simulink library "PowerFlowLib2013amdl"  (Simulink 8.1)
settings: Solver=ode45  StartTime=0.0  StopTime=10.0  RelTol=1e-3
undefined symbols (not defined in the file or in its folder): AirProp, C, F1, Fanmap, Fld1, Fld2, fueltankdata, HydProp, HydraulicLoad, IBFD_exc, L, LoadFluidProps, magnitude, MSSN, n_alghts, PumpProp, pwr_alghts, R_fd_exc, Rcore, Ts, VBFD_exc
libraries: PowerFlowLib x32, simulink x14, powerlib_extras x2, dspstat3 x2
(part 4 of 11)

== system PowerFlowLib2013amdl/Energy & Power Systems/Additional Systems ==
  Commercial Cabin Systems : Subsystem  mask(Commercial Cabin Systems){n_pax=150, n_sockets=3, n_oven=4, pwr_oven=3800, pf_oven=.707, q_oven=95, n_bev=3, pwr_bev=3800, pf_bev=.707, q_bev=95, n_rlghts=150, pwr_rlghts=5, q_rlghts=95, n_clghts=20, pwr_clghts=15, q_clghts=95, n_IFE=150, pwr_IFE=25}
      mask prompts: n_pax "Seating Capacity"; n_sockets "Number of Electrical Sockets in Cabin"; n_oven "Number of Ovens"; pwr_oven "Nominal Power [W]"; pf_oven "Power Factor"; q_oven "Heat Loss Output [W]"; n_bev "Number of Beverage Makers"; pwr_bev "Nominal Power [W]"; pf_bev "Power Factor"; q_bev "Heat Loss Output [W]"; n_rlghts "Number of Reading Lights"; pwr_rlghts "Power Consumption per Lamp [W]"; q_rlghts "Heat Loss Output [W]"; n_clghts "Number of Cabin Lights"; pwr_clghts "Power Consumption per Light [W]"; q_clghts "Heat Loss Output [W]"; n_IFE "Individual Seat Models"; pwr_IFE "Power Consumption per Seat Model [W]"
      mask help:
      | Calculation of galley electrical loads, cabin lighting loads, and in-flight entertainment (IFE) electrical loads.
      |
      | Input to the block requires the mission profile for determination of usage and cyclical loading.
  External Lights : Subsystem  mask(Commercial Cabin Systems){n_pax=150, n_sockets=3, n_oven=4, pwr_oven=3800, pf_oven=.707, q_oven=95, n_bev=3, pwr_bev=3800, pf_bev=.707, q_bev=95, n_rlghts=150, pwr_rlghts=5, q_rlghts=95, n_clghts=20, pwr_clghts=15, q_clghts=95, n_IFE=150, pwr_IFE=25}
      mask prompts: n_pax "Seating Capacity"; n_sockets "Number of Electrical Sockets in Cabin"; n_oven "Number of Ovens"; pwr_oven "Nominal Power [W]"; pf_oven "Power Factor"; q_oven "Heat Loss Output [W]"; n_bev "Number of Beverage Makers"; pwr_bev "Nominal Power [W]"; pf_bev "Power Factor"; q_bev "Heat Loss Output [W]"; n_rlghts "Number of Reading Lights"; pwr_rlghts "Power Consumption per Lamp [W]"; q_rlghts "Heat Loss Output [W]"; n_clghts "Number of Cabin Lights"; pwr_clghts "Power Consumption per Light [W]"; q_clghts "Heat Loss Output [W]"; n_IFE "Individual Seat Models"; pwr_IFE "Power Consumption per Seat Model [W]"
      mask help:
      | Calculation of galley electrical loads, cabin lighting loads, and in-flight entertainment (IFE) electrical loads.
      |
      | Input to the block requires the mission profile for determination of usage and cyclical loading.

== system PowerFlowLib2013amdl/Energy & Power Systems/Electrical ==
  Battery : Subsystem
  Converters : Subsystem
  Coordinate Transformation : Subsystem
  Inverters : Subsystem
  Loads : Subsystem
  Loss Estimation : Subsystem
  Machines : Subsystem
  Rectifiers : Subsystem
  Systems : Subsystem

== system PowerFlowLib2013amdl/Energy & Power Systems/Hydraulic ==
  Bypass Valve : Subsystem  mask(Bypass Valve){}
      mask help:
      | Calculates hydraulic fluid bypass.
      |
      | Flow Out - hydraulic fluid flow to the actuators.
      | Bypass - hydraulic fluid flow back to the reservoir.
      mask Display:
      | port_label('input',1,'{\bf Flow In}','TexMode','on')
      | port_label('input',2,'{\bf Req Flow}','TexMode','on')
      | 
      | port_label('output',1,'{\bf Flow Out}','TexMode','on')
      | port_label('output',2,'{\bf Bypass}','TexMode','on')
  Engine Driven Pump : Subsystem  mask(Engine Driven Hydraulic Pump){RPM=3750, disp=39, eta_mech=95, eta_v=85, nom_T=40, nom_w=393, nom_delP=20684}
      mask prompts: RPM "Fixed RPM"; disp "Fixed Displacement [cm³/rev]"; eta_mech "Mechanical Efficiency [%]"; eta_v "Volumetric Efficiency [%]"; nom_T "Nominal Fluid Temperature [°C]"; nom_w "Nominal Angular Velocity [rad/s]"; nom_delP "Nominal Pressure Differential [kPa]"
      mask help:
      | This is a fixed displacement, uni-directional hydraulic pump.  Flow rate is calculated by this block.  Pressure up-stream and down-stream are required inputs.
      |
      | Block Inputs
      | #1: Hydraulic fluid properties from reservoir
      | #2: Shaft RPM from aux. gear box
      | #3: Upstream system hydraulic pressure [kPa]
      |
      | Block Outputs
      | #1: Fluid properties
      | #2: Shaft torque applied to aux. gear box [Nm]
      mask Callback eta_mech:
      | h      = get_param(gcb,'handle');   % Get block handle
      | hblock = get(h);                    % Parse out handles structure
      | 
      | if str2num(hblock.eta_mech) == 0
      |     set_param(gcb,'eta_mech','100')
      | elseif str2num(hblock.eta_mech) < 1
      |     set_param(gcb,'eta_mech',num2str(str2num(hblock.eta_mech)*100))
      | elseif str2num(hblock.eta_mech) > 100
      |     set_param(gcb,'eta_mech',num2str(100))
      | end
      | 
      | clear h hblock
      mask Callback eta_v:
      | h      = get_param(gcb,'handle');   % Get block handle
      | hblock = get(h);                    % Parse out handles structure
      | 
      | if str2num(hblock.eta_v) == 0
      |     set_param(gcb,'eta_v','100')
      | elseif str2num(hblock.eta_v) < 1
      |     set_param(gcb,'eta_v',num2str(str2num(hblock.eta_v)*100))
      | elseif str2num(hblock.eta_v) > 100
      |     set_param(gcb,'eta_v',num2str(100))
      | end
      | 
      | clear h hblock
      mask Display:
      | image(imread('hyd_edp_fixed.png'))
      | 
      | port_label('input',1,'{\bf Flow In}','TexMode','on')
      | port_label('input',2,'{\bf Shaft RPM}','TexMode','on')
      | port_label('input',3,'{\bf System Pressure (kPa)}','TexMode','on')
      | 
      | port_label('output',1,'{\bf Flow Out}','TexMode','on')
      | port_label('output',2,'{\bf Shaft Torque (Nm)}','TexMode','on')
  Fluid Reservoir : Subsystem  mask(Fluid Reservoir){res_vol=.25, bleed_flowrate=.05, pres_loss=1, T_init=300, P_init=1500, mass_init=30}
      mask prompts: res_vol "Resevoir Volume [m³]"; bleed_flowrate "Max Bleed Air Supply Rate [kg/s]"; pres_loss "Air Pressure Losses [%]"; T_init "Initial Fluid Temp [K]"; P_init "Initial Air Pressure [kPa]"; mass_init "Initial Fluid Mass [kg]"
      mask help:
      | Block Inputs
      | #1: Bleed air properties (Bus signal)
      | #2: Bypass return from bypass valve
      | #3: Mass flow rate pumped out by hydraulic pump
      | #4: Mass flow rate returned from actuators
      |
      | Block Outputs
      | #1: Bleed air demanded to maintain pressurization
      | #2: Hydraulic fluid properties in the reservoir
      mask Display:
      | image(imread('hyd_res.png'))
      | 
      | port_label('input',1,'{\bf Bleed In}','TexMode','on')
      | port_label('input',2,'{\bf Bypass Return}','TexMode','on')
      | port_label('input',3,'{\bf m_d_o_t Out}','TexMode','on')
      | port_label('input',4,'{\bf m_d_o_t Return}','TexMode','on')
      | 
      | port_label('output',1,'{\bf Bleed Demand}','TexMode','on')
      | port_label('output',2,'{\bf Fluid Out}','TexMode','on')
  Hydraulic Load : Subsystem  mask(Hydraulic Loading){fileslct=off, filename=HydraulicLoad.mat, filedir=C:\Users\mwillms4\Dropbox\School\Graduate\Research\PowerFlow Development\PowerFlow Summer 2013\PropertyTables\HydraulicLoad.mat, var_struct=HydraulicLoad, h_load=B_737 - rudder}
      mask prompts: fileslct "Select Hydraulic Load File?"; filename "Hydraulic Load File"; filedir "Hydraulic Load File Location"; var_struct "Structure Name (in workspace)"; h_load "Hydraulic Load"
      mask init:
      | h      = get_param(gcb,'handle');   % Get block handle
      | blk    = gcb; 
      | hblock = get(h);
      | 
      | set_param(blk,'fileslct','off');     % turn off manual switch
      | 
      | [platform,load] = strtok(hblock.h_load,' - ');
      | set_param([blk,'/m_dot'],'Table',[hblock.var_struct,'.',platform,'.',load(4:size(load,2))]);
      | 
      | [a,b] = size(evalin('base',[hblock.var_struct,'.',platform,'.',load(4:size(load,2))]));
      | 
      | set_param([blk,'/m_dot'],'BreakpointsForDimension1',['[1:',num2str(a),']']);
      | set_param([blk,'/m_dot'],'BreakpointsForDimension2',['[0:',num2str(b-1),']']);
      | 
      | clear h blk hblock a b platform load
      mask Callback fileslct:
      | h      = get_param(gcb,'handle');   % Get block handle
      | blk    = gcb;
      | hblock = get(h);     % Parse out handles structure
      | 
      | 
      | if strcmp(hblock.fileslct,'on') == 1;
      |     RR_SetPerfSlct(2,0);                    % call uiopen script
      |     set_param(blk,'fileslct','off');     % turn off manual switch
      | 
      |     hblock = get(h);
      | 
      |     s = whos('-FILE',hblock.filedir);
      |     if exist(s.name) == 1
      |         error(['Variable ',s.name,' already exists in the Workspace. Unable to load ',hblock.filename])
      |     end
      | end
      | 
      | clear h blk hblock s
      mask TypeOptions h_load: B_737 - rudder | B_737 - ailerons | B_737 - landing_gear | B_737 - elevator | B_737 - thrust_rev | Emb_145 - rudder | Emb_145 - ailerons | Emb_145 - landing_gear | Emb_145 - elevator | Emb_145 - thrust_rev
      mask Callback h_load:
      | h      = get_param(gcb,'handle');   % Get block handle
      | blk    = gcb;
      | hblock = get(h);     % Parse out handles structure
      | 
      | if strcmp('0',hblock.filename) ~= 1
      |     s = whos('-FILE',hblock.filename);
      | 
      |     while strcmp('<no load>',hblock.h_load) == 1
      | 
      |         hydr = fieldnames(eval(s.name));
      |         for i = 1:size(hydr,1)
      |             hydr_load = fieldnames(getfield(HydraulicLoad,hydr{i}));
      |             for j = 1:size(hydr_load,1);
      |                if ((j==1) && (i==1))
      |                     hydstr_ld = [hydr{i},' - ',hydr_load{j}];
      |                else
      |                     hydstr_ld = strcat(hydstr_ld,char(124),[hydr{i},' - ',hydr_load{j}]);
      |                end
      |             end
      |         end
      | 
      |         % Get the mask parameter values. This is a cell array of strings.
      |         styl = get_param(blk,'MaskStyles');
      |         vis = get_param(blk,'MaskVisibilities');
      |         str = get_param(blk,'MaskPromptString');
      | 
      |         % fill the mask with the parameters
      |         set_param(blk,'MaskVisibilities',vis,'MaskPromptString',str,'MaskStyles',[styl(1:3);strcat('popup(',hydstr_ld,')');styl(5)]);
      | 
      |         hblock = get(h);     % Parse out handles structure
      |     end
      | 
      | 
      | end
      | clear s h blk hblock styl vals vis str pmpstr i indx pumps hydstr hydr j
      mask Display:
      | port_label('input',1,'{\bf Flow In}','TexMode','on')
      | port_label('input',2,'{\bf Flight Phase}','TexMode','on')
      | 
      | port_label('output',1,'{\bf Return}','TexMode','on')
      | port_label('output',2,'{\bf Power}','TexMode','on')
      | 
      | text(0.5,0.9,get_param(gcb,'h_load'),'horizontalAlignment','center')

== system PowerFlowLib2013amdl/Energy & Power Systems/Thermal ==
  Anti-Ice : Subsystem  mask(Anti-Ice System){ice_sys=Wing, E_src=Electrical, dfine=off, pwr=0, m_dot=0}
      mask prompts: ice_sys "Anti-Ice System"; E_src "Energy Source"; dfine "Define Energy Consumption Externally?"; pwr "Power Consumption [kW]"; m_dot "Bleed Air Flow Rate [kg/s]"
      mask help:
      | Simulates power lost due to anti-ice systems.
      |
      | Block Inputs:
      | 1. On/Off Control Input (1/0 for On/Off)
      | 2. Power/Flow Rate Consumption (optional)
      | Note: Keep units as kg/s or kW
      |
      | Block Outputs:
      | 1. Demanded Electrical Power or Mass Flow Rate
      mask init:
      | h      = get_param(gcb,'handle');   % Get block handle
      | blk    = gcb; 
      | hblock = get(h);     % Parse out handles structure 
      | 
      | if strcmp('on',hblock.dfine) == 1;
      |     
      | else
      |     
      |     if strcmp('Engine Bleed Air',hblock.E_src) == 1;
      |         set_param([gcb,'/Load'],'Value',hblock.m_dot)
      |     elseif strcmp('APU Bleed Air',hblock.E_src) == 1;
      |         set_param([gcb,'/Load'],'Value',hblock.m_dot)
      |     elseif strcmp('Pneumatic Manifold',hblock.E_src) == 1;
      |         set_param([gcb,'/Load'],'Value',hblock.m_dot)
      |     elseif strcmp('Electrical',hblock.E_src) == 1;
      |         set_param([gcb,'/Load'],'Value',hblock.pwr)
      |     else
      |         msgbox(['Incorrect setting for Energy Source in ',hblock.Name]);
      |     end
      |         
      | end
      | 
      | 
      | try
      |     delete_line(blk,'LoadSwitch/1','LoadBus/1');
      | end
      | 
      | linehandle = add_line(blk,'LoadSwitch/1','LoadBus/1');
      | 
      | if strcmp('Engine Bleed Air',hblock.E_src) == 1;
      |     set(linehandle,'name','mdot_kgps');
      | elseif strcmp('APU Bleed Air',hblock.E_src) == 1;
      |     set(linehandle,'name','mdot_kgps');
      | elseif strcmp('Pneumatic Manifold',hblock.E_src) == 1;
      |     set(linehandle,'name','mdot_kgps');
      | elseif strcmp('Electrical',hblock.E_src) == 1;
      |     set(linehandle,'name','pwr_kW');
      | else
      |     msgbox(['Incorrect setting for Energy Source in ',hblock.Name]);
      | end
      | 
      | 
      | 
      | 
      | clear h blk hblock
      mask TypeOptions ice_sys: Engine Cowl | Wing
      mask TypeOptions E_src: Engine Bleed Air | APU Bleed Air | Pneumatic Manifold | Electrical
      mask Callback E_src:
      | h      = get_param(gcb,'handle');   % Get block handle
      | blk    = gcb;
      | hblock = get(h);     % Parse out handles structure
      | 
      | vis = get_param(blk,'MaskVisibilities');
      | if strcmp('on',hblock.dfine) == 0;
      |     if strcmp('Engine Bleed Air',hblock.E_src) == 1;
      |         set_param(blk,'MaskVisibilities',{vis{1};vis{2};vis{3};'off';'on'}) % set visibility
      |     elseif strcmp('APU Bleed Air',hblock.E_src) == 1;
      |         set_param(blk,'MaskVisibilities',{vis{1};vis{2};vis{3};'off';'on'}) % set visibility
      |     elseif strcmp('Pneumatic Manifold',hblock.E_src) == 1;
      |         set_param(blk,'MaskVisibilities',{vis{1};vis{2};vis{3};'off';'on'}) % set visibility
      |     elseif strcmp('Electrical',hblock.E_src) == 1;
      |         set_param(blk,'MaskVisibilities',{vis{1};vis{2};vis{3};'on';'off'}) % set visibility
      |     else
      |         msgbox(['Incorrect setting for Energy Source in ',hblock.Name]);
      |     end
      | end
      | 
      | clear h blk hblock vis
      mask Callback dfine:
      | h      = get_param(gcb,'handle');   % Get block handle
      | blk    = gcb;
      | hblock = get(h);     % Parse out handles structure
      | 
      | vis = get_param(blk,'MaskVisibilities');
      | 
      | if strcmp('on',hblock.dfine) == 1;
      |     try
      |         add_block('simulink/Sources/In1',[blk,'/Value'],'Position',[30,30,60,43]);
      |         delete_unconnected_lines();
      |         add_line(blk,'Value/1','Switch1/1');
      |     end
      |     set_param([blk,'/External Define'],'Value','1');
      |     set_param(blk,'MaskVisibilities',{vis{1};vis{2};vis{3};'off';'off'})
      | else
      |     set_param([blk,'/External Define'],'Value','0');
      |     try
      |         delete_block([blk,'/Value']);
      |     end
      |     if strcmp('Engine Bleed Air',hblock.E_src) == 1;
      |         set_param(blk,'MaskVisibilities',{vis{1};vis{2};vis{3};'off';'on'}) % set visibility
      |     elseif strcmp('APU Bleed Air',hblock.E_src) == 1;
      |         set_param(blk,'MaskVisibilities',{vis{1};vis{2};vis{3};'off';'on'}) % set visibility
      |     elseif strcmp('Pneumatic Manifold',hblock.E_src) == 1;
      |         set_param(blk,'MaskVisibilities',{vis{1};vis{2};vis{3};'off';'on'}) % set visibility
      |     elseif strcmp('Electrical',hblock.E_src) == 1;
      |         set_param(blk,'MaskVisibilities',{vis{1};vis{2};vis{3};'on';'off'}) % set visibility
      |     else
      |         msgbox(['Incorrect setting for Energy Source in ',hblock.Name]);
      |     end
      | end
      | 
      | clear h blk hblock vis
      mask Display:
      | h      = get_param(gcb,'handle');   % Get block handle
      | blk    = gcb;
      | hblock = get(h);     % Parse out handles structure
      | 
      | text(0.5,0.9,['Source: ',hblock.E_src],'HorizontalAlignment','center')
      | 
      | port_label('input',1,'{\bf Control}','TexMode','on')
      | 
      | if strcmp('Engine Bleed Air',hblock.E_src) == 1;
      |     port_label('output',1,'{\bf Bleed Air Demand}','TexMode','on')
      | elseif strcmp('APU Bleed Air',hblock.E_src) == 1;
      |     port_label('output',1,'{\bf Bleed Air Demand}','TexMode','on')
      | elseif strcmp('Pneumatic Manifold',hblock.E_src) == 1;
      |     port_label('output',1,'{\bf Bleed Air Demand}','TexMode','on')
      | elseif strcmp('Electrical',hblock.E_src) == 1;
      |     port_label('output',1,'{\bf Elec Pwr Demand}','TexMode','on')
      | else
      |     msgbox(['Incorrect setting for Energy Source in ',hblock.Name]);
      | end
      | 
      | if strcmp('on',hblock.dfine) == 1;
      |     port_label('input',2,'{\bf Value}','TexMode','on')
      | end
      | 
      | clear h blk hblock
  ECS : Subsystem
  Fuel & Oil : Subsystem

== system PowerFlowLib2013amdl/Mission Profile/Mission Profile ==
  APU : Lookup  InputValues=MSSN.eng.time  Table=MSSN.eng.apu  LookUpMeth=Use Input Below
  Add : Sum
  Add1 : Sum
  Add2 : Sum
  Alt : Lookup  InputValues=MSSN.cond.time  Table=MSSN.cond.alt
  Bus Creator1 : BusCreator  Inputs=3
  Bus Creator2 : BusCreator
  Bus Creator3 : BusCreator
  Bus Creator4 : BusCreator  Inputs=5
  Clock : Clock
  Constant1 : Constant  Value=del_T
  Constant2 : Constant  Value=del_P
  Constant3 : Constant  Value=del_rho
  Engine 1 : Lookup  InputValues=MSSN.eng.time  Table=MSSN.eng.Eng1  LookUpMeth=Use Input Below
  Engine 2 : Lookup  InputValues=MSSN.eng.time  Table=MSSN.eng.Eng2  LookUpMeth=Use Input Below
  Flaps : Lookup  InputValues=MSSN.el.time  Table=MSSN.el.flaps  LookUpMeth=Use Input Below
  Gain : Gain  Gain=temp_msl + 273.15
  Gain1 : Gain  Gain=pres_msl
  Gain2 : Gain  Gain=dens_msl
  Landing lights : Lookup  InputValues=MSSN.el.time  Table=MSSN.el.landinglit  LookUpMeth=Use Input Below
  Mach : Lookup  InputValues=MSSN.cond.time  Table=MSSN.cond.mach
  Mssn Phase : Lookup  InputValues=MSSN.gen.time  Table=MSSN.gen.state  LookUpMeth=Use Input Below
  Pressurization : Lookup  InputValues=MSSN.pnu.time  Table=MSSN.pnu.pres  LookUpMeth=Use Input Below
  Taxi Lights : Lookup  InputValues=MSSN.el.time  Table=MSSN.el.taxilit  LookUpMeth=Use Input Below
  delta (P/P0) : Lookup_n-D  NumberOfTableDimensions=1  BreakpointsForDimension1=|  Table=|  RndMeth=Simplest  InputSameDT=on
      BreakpointsForDimension1=|
      | [0
      | 1000
      | 2000
      | 3000
      | 4000
      | 5000
      | 6000
      | 7000
      | 8000
      | 9000
      | 10000
      | 11000
      | 12000
      | 13000
      | 14000
      | 15000
      | 16000
      | 17000
      | 18000
      | 19000
      | 20000
      | 21000
      | 22000
      | 23000
      | 24000
      | 25000
      | 26000
      | 27000
      | 28000
      | 29000
      | 30000
      | 31000
      | 32000
      | 33000
      | 34000
      | 35000
      | 36000
      | 37000
      | 38000
      | 39000
      | 40000
      | 41000
      | 42000
      | 43000
      | 44000
      | 45000
      | 46000
      | 47000
      | 48000
      | 49000
      | 50000
      | 51000
      | 52000
      | 53000
      | 54000
      | 55000
      | 56000
      | 57000
      | 58000
      | 59000
      | 60000
      | 61000
      | 62000
      | 63000
      | 64000
      | 65000
      | ]
      Table=|
      | [1
      | 0.9644
      | 0.9298
      | 0.8963
      | 0.8637
      | 0.8321
      | 0.8014
      | 0.7717
      | 0.7429
      | 0.7149
      | 0.6878
      | 0.6616
      | 0.6362
      | 0.6115
      | 0.5877
      | 0.5646
      | 0.5422
      | 0.5206
      | 0.4997
      | 0.4795
      | 0.4599
      | 0.441
      | 0.4227
      | 0.4051
      | 0.388
      | 0.3716
      | 0.3557
      | 0.3404
      | 0.3256
      | 0.3113
      | 0.2975
      | 0.2843
      | 0.2715
      | 0.2592
      | 0.2474
      | 0.236
      | 0.225
      | 0.2145
      | 0.2044
      | 0.1949
      | 0.1858
      | 0.1771
      | 0.1688
      | 0.1609
      | 0.1534
      | 0.1462
      | 0.1394
      | 0.1329
      | 0.1267
      | 0.1208
      | 0.1151
      | 0.1097
      | 0.1046
      | 0.0997
      | 0.0951
      | 0.0906
      | 0.0864
      | 0.0824
      | 0.0785
      | 0.0749
      | 0.0714
      | 0.068
      | 0.0649
      | 0.0618
      | 0.059
      | 0.0562
      | 
      | 
      | ]
  sigma (rho/rho-0) : Lookup_n-D  NumberOfTableDimensions=1  BreakpointsForDimension1=|  Table=|  RndMeth=Simplest  InputSameDT=on
      BreakpointsForDimension1=|
      | [0
      | 1000
      | 2000
      | 3000
      | 4000
      | 5000
      | 6000
      | 7000
      | 8000
      | 9000
      | 10000
      | 11000
      | 12000
      | 13000
      | 14000
      | 15000
      | 16000
      | 17000
      | 18000
      | 19000
      | 20000
      | 21000
      | 22000
      | 23000
      | 24000
      | 25000
      | 26000
      | 27000
      | 28000
      | 29000
      | 30000
      | 31000
      | 32000
      | 33000
      | 34000
      | 35000
      | 36000
      | 37000
      | 38000
      | 39000
      | 40000
      | 41000
      | 42000
      | 43000
      | 44000
      | 45000
      | 46000
      | 47000
      | 48000
      | 49000
      | 50000
      | 51000
      | 52000
      | 53000
      | 54000
      | 55000
      | 56000
      | 57000
      | 58000
      | 59000
      | 60000
      | 61000
      | 62000
      | 63000
      | 64000
      | 65000
      | ]
      Table=|
      | [1
      | 0.9711
      | 0.9428
      | 0.9151
      | 0.8881
      | 0.8617
      | 0.8359
      | 0.8107
      | 0.7861
      | 0.7621
      | 0.7386
      | 0.7157
      | 0.6933
      | 0.6715
      | 0.6502
      | 0.6295
      | 0.6092
      | 0.5895
      | 0.5702
      | 0.5514
      | 0.5332
      | 0.5153
      | 0.498
      | 0.4811
      | 0.4646
      | 0.4486
      | 0.433
      | 0.4178
      | 0.4031
      | 0.3887
      | 0.3747
      | 0.3611
      | 0.348
      | 0.3351
      | 0.3227
      | 0.3106
      | 0.2988
      | 0.2852
      | 0.2719
      | 0.2592
      | 0.2471
      | 0.2355
      | 0.2245
      | 0.214
      | 0.204
      | 0.1945
      | 0.1854
      | 0.1767
      | 0.1685
      | 0.1606
      | 0.1531
      | 0.146
      | 0.1391
      | 0.1326
      | 0.1264
      | 0.1205
      | 0.1149
      | 0.1096
      | 0.1044
      | 0.0996
      | 0.0949
      | 0.0905
      | 0.0863
      | 0.0822
      | 0.0784
      | 0.0747
      | 
      | ]
  theta (T/T0) : Lookup_n-D  NumberOfTableDimensions=1  BreakpointsForDimension1=|  Table=|  RndMeth=Simplest  InputSameDT=on
      BreakpointsForDimension1=|
      | [0
      | 1000
      | 2000
      | 3000
      | 4000
      | 5000
      | 6000
      | 7000
      | 8000
      | 9000
      | 10000
      | 11000
      | 12000
      | 13000
      | 14000
      | 15000
      | 16000
      | 17000
      | 18000
      | 19000
      | 20000
      | 21000
      | 22000
      | 23000
      | 24000
      | 25000
      | 26000
      | 27000
      | 28000
      | 29000
      | 30000
      | 31000
      | 32000
      | 33000
      | 34000
      | 35000
      | 36000
      | 37000
      | 38000
      | 39000
      | 40000
      | 41000
      | 42000
      | 43000
      | 44000
      | 45000
      | 46000
      | 47000
      | 48000
      | 49000
      | 50000
      | 51000
      | 52000
      | 53000
      | 54000
      | 55000
      | 56000
      | 57000
      | 58000
      | 59000
      | 60000
      | 61000
      | 62000
      | 63000
      | 64000
      | 65000
      | ]
      Table=|
      | [1
      | 0.9931
      | 0.9863
      | 0.9794
      | 0.9725
      | 0.9656
      | 0.9588
      | 0.9519
      | 0.945
      | 0.9381
      | 0.9313
      | 0.9244
      | 0.9175
      | 0.9107
      | 0.9038
      | 0.8969
      | 0.8901
      | 0.8832
      | 0.8763
      | 0.8695
      | 0.8626
      | 0.8558
      | 0.8489
      | 0.842
      | 0.8352
      | 0.8283
      | 0.8215
      | 0.8146
      | 0.8077
      | 0.8009
      | 0.794
      | 0.7872
      | 0.7803
      | 0.7735
      | 0.7666
      | 0.7598
      | 0.7529
      | 0.7519
      | 0.7519
      | 0.7519
      | 0.7519
      | 0.7519
      | 0.7519
      | 0.7519
      | 0.7519
      | 0.7519
      | 0.7519
      | 0.7519
      | 0.7519
      | 0.7519
      | 0.7519
      | 0.7519
      | 0.7519
      | 0.7519
      | 0.7519
      | 0.7519
      | 0.7519
      | 0.7519
      | 0.7519
      | 0.7519
      | 0.7519
      | 0.7519
      | 0.7519
      | 0.7519
      | 0.7519
      | 0.7519
      | 
      | ]
  Mission Parameters : Outport
  wires:
  Clock/1 -> Pressurization/1, Flaps/1, Landing lights/1, Taxi Lights/1, APU/1, Engine 2/1, Engine 1/1, Mssn Phase/1, Mach/1, Alt/1
  Engine 1/1 -> Bus Creator1/1  "E_1"
  Engine 2/1 -> Bus Creator1/2  "E_2"
  Bus Creator1/1 -> Bus Creator2/3  "Engines"
  Bus Creator3/1 -> Bus Creator2/4  "Mission Misc"
  Taxi Lights/1 -> Bus Creator3/1  "T_light"
  APU/1 -> Bus Creator1/3  "apu"
  Landing lights/1 -> Bus Creator3/2  "L_light"
  Pressurization/1 -> Bus Creator3/3  "Pres_on/off"
  Flaps/1 -> Bus Creator3/4  "Flapset"
  Mssn Phase/1 -> Bus Creator2/2  "Mssn_phase"
  Alt/1 -> delta (P/P0)/1, sigma (rho/rho-0)/1, theta (T/T0)/1, Bus Creator4/4  "altitude_ft"
  Constant1/1 -> Add/2
  Constant2/1 -> Add1/2
  Constant3/1 -> Add2/2
  Gain2/1 -> Add2/1  "std_dens_kg/m3"
  Gain1/1 -> Add1/1  "std_pres_kPa"
  Gain/1 -> Add/1  "std_temp_K"
  theta (T/T0)/1 -> Gain/1
  sigma (rho/rho-0)/1 -> Gain2/1
  delta (P/P0)/1 -> Gain1/1
  Add2/1 -> Bus Creator4/1  "rho_kgpm3"
  Add1/1 -> Bus Creator4/2  "pres_kPa"
  Add/1 -> Bus Creator4/3  "temp_K"
  Mach/1 -> Bus Creator4/5  "Mach"
  Bus Creator4/1 -> Bus Creator2/1  "Flight parameters"
  Bus Creator2/1 -> Mission Parameters/1

== system PowerFlowLib2013amdl/Support Functions/Tools/ElectricalSink ==
  Load In : Inport
  React. Pwr : Inport  Port=2
  Sum of Elements : Sum  Inputs=+
  loadsbus : BusCreator  Inputs=2
  units : Gain  Gain=1000
  tag scope: Cockpit_ElecAC_8332=global
  wires:
  Load In/1 -> Sum of Elements/1  "Inlet"
  Sum of Elements/1 -> loadsbus/1  "real_pwr_W"
  loadsbus/1 -> units/1
  units/1 -> [Cockpit_ElecAC_8332]
  React. Pwr/1 -> loadsbus/2  "react_pwr"

== system PowerFlowLib2013amdl/Support Functions/Tools/ElectricalSource ==
  LoadBus : BusCreator  Inputs=1
  Load : Outport
  wires:
  LoadBus/1 -> Load/1

== system PowerFlowLib2013amdl/Support Functions/Tools/FluidComponent Properties ==

== system PowerFlowLib2013amdl/Support Functions/Tools/PowerFlow Data Manager ==
  Data : Outport

== system PowerFlowLib2013amdl/Support Functions/Tools/ThermalSink ==
  Flow In : Inport
  Sum of Elements : Sum  Inputs=+
  units : Gain  Gain=1000
  tag scope: Cabin_Therm_9151=global
  wires:
  Flow In/1 -> units/1  "Inlet"
  Sum of Elements/1 -> [Cabin_Therm_9151]  "heatloads_W"
  units/1 -> Sum of Elements/1

== system PowerFlowLib2013amdl/Support Functions/Tools/ThermalSource ==
  LoadBus : BusCreator
  Load : Outport
  wires:
  LoadBus/1 -> Load/1

== system PowerFlowLib2013amdl/Support Functions/Tools/Unit Conversion  ==
  Signal_in : Inport
  conv_fcn : Fcn  Expr=(u(1)+273.15)-273.15
  Converted Signal Out : Outport
  wires:
  conv_fcn/1 -> Converted Signal Out/1
  Signal_in/1 -> conv_fcn/1

== system PowerFlowLib2013amdl/Support Functions/Tools/data_sink ==
  " " : Inport
  tag scope: gdata_PowerFlowLibSupportFunctionsToolsdata_sink=global
  wires:
  " "/1 -> [gdata_PowerFlowLibSupportFunctionsToolsdata_sink]

== system PowerFlowLib2013amdl/Energy & Power Systems/Additional Systems/Commercial Cabin Systems ==
  Mission : Inport
  (1-pf)/pf : Gain  Gain=(1-pf_oven)/(pf_oven+eps)
  (1-pf)/pf1 : Gain  Gain=(1-pf_bev)/(pf_bev+eps)
  Bus Creator : BusCreator  Inputs=3
  Bus Creator1 : BusCreator  Inputs=3
  Bus Creator2 : BusCreator  Inputs=5
  Bus Creator3 : BusCreator  Inputs=2
  Bus Creator4 : BusCreator  Inputs=2
  Bus Creator5 : BusCreator  Inputs=1
  Bus Selector : BusSelector  OutputSignals=GalleyOvens_on/off
  Bus Selector1 : BusSelector  OutputSignals=GalleyBev_on/off
  Bus Selector2 : BusSelector  OutputSignals=ReadingLights_%on
  Bus Selector3 : BusSelector  OutputSignals=CabinLights_%on
  Bus Selector4 : BusSelector  OutputSignals=IFEmodules_%on
  Constant : Constant  Value=n_oven*pwr_oven
  Constant1 : Constant  Value=n_bev*pwr_bev
  Constant2 : Constant  Value=n_rlghts * pwr_rlghts
  Constant3 : Constant  Value=n_alghts * pwr_alghts
  Constant4 : Constant  Value=n_IFE * pwr_IFE
  Constant5 : Constant  Value=q_oven
  Constant6 : Constant  Value=q_bev
  Constant7 : Constant  Value=q_rlghts
  Constant8 : Constant  Value=q_clghts
  ElectricalSink : PowerFlowLib/Support Functions//Tools/ElectricalSink  Tag=Flow  Description=TwoPhase  load_loc=Cabin  ACDC_load=AC  units=Watts  unq_id=8332
  ElectricalSink1 : PowerFlowLib/Support Functions//Tools/ElectricalSink  Tag=Flow  Description=TwoPhase  load_loc=Cabin  ACDC_load=AC  units=Watts  unq_id=9151
  ElectricalSink2 : PowerFlowLib/Support Functions//Tools/ElectricalSink  Tag=Flow  Description=TwoPhase  load_loc=Cabin  ACDC_load=DC  units=Watts  unq_id=2143
  ElectricalSink3 : PowerFlowLib/Support Functions//Tools/ElectricalSink  Tag=Flow  Description=TwoPhase  load_loc=Cabin  ACDC_load=DC  units=Watts  unq_id=9219
  ElectricalSink4 : PowerFlowLib/Support Functions//Tools/ElectricalSink  Tag=Flow  Description=TwoPhase  load_loc=Cabin  ACDC_load=DC  units=Watts  unq_id=6691
  Product{,1..4} (5 alike) : Product  RndMeth=Zero
  ThermalSink : PowerFlowLib/Support Functions//Tools/ThermalSink  Tag=Flow  Description=TwoPhase  load_loc=Cabin  units=Watts  unq_id=1878
  ThermalSink1 : PowerFlowLib/Support Functions//Tools/ThermalSink  Tag=Flow  Description=TwoPhase  load_loc=Cabin  units=Watts  unq_id=3506
  ThermalSink2 : PowerFlowLib/Support Functions//Tools/ThermalSink  Tag=Flow  Description=TwoPhase  load_loc=Cabin  units=Watts  unq_id=5921
  ThermalSink3 : PowerFlowLib/Support Functions//Tools/ThermalSink  Tag=Flow  Description=TwoPhase  load_loc=Cabin  units=Watts  unq_id=9617
  data_sink : PowerFlowLib/Support Functions//Tools/data_sink
  wires:
  (1-pf)/pf/1 -> ElectricalSink/2, Bus Creator/3  "react_pwr_VAr"
  Constant/1 -> Product/1
  Product/1 -> (1-pf)/pf/1, ElectricalSink/1, Bus Creator/2  "real_pwr_W"
  (1-pf)/pf1/1 -> ElectricalSink1/2, Bus Creator1/2  "react_pwr_VAr"
  Constant1/1 -> Product1/1
  Product1/1 -> (1-pf)/pf1/1, ElectricalSink1/1, Bus Creator1/1  "real_pwr_W"
  Constant2/1 -> Product2/1
  Product2/1 -> ElectricalSink2/1, Bus Creator3/1  "pwr_W"
  Constant3/1 -> Product3/1
  Product3/1 -> ElectricalSink3/1, Bus Creator4/2  "pwr_W"
  Constant4/1 -> Product4/1
  Product4/1 -> ElectricalSink4/1, Bus Creator5/1  "pwr_W"
  Mission/1 -> Bus Selector/1, Bus Selector1/1, Bus Selector2/1, Bus Selector4/1, Bus Selector3/1
  Bus Selector4/1 -> Product4/2  "<IFEmodules_%on>"
  Bus Selector3/1 -> Product3/2  "<CabinLights_%on>"
  Bus Selector2/1 -> Product2/2  "<ReadingLights_%on>"
  Bus Selector1/1 -> Product1/2  "<GalleyBev_on/off>"
  Bus Selector/1 -> Product/2  "<GalleyOvens_on/off>"
  Bus Creator2/1 -> data_sink/1
  Bus Creator/1 -> Bus Creator2/1  "Ovens"
  Bus Creator1/1 -> Bus Creator2/2  "Bev_Makers"
  Bus Creator3/1 -> Bus Creator2/3  "ReadLights"
  Bus Creator4/1 -> Bus Creator2/4  "CabLights"
  Bus Creator5/1 -> Bus Creator2/5  "IFE"
  Constant5/1 -> ThermalSink/1, Bus Creator/1  "heat_W"
  Constant6/1 -> ThermalSink1/1, Bus Creator1/3  "heat_W"
  Constant7/1 -> ThermalSink2/1, Bus Creator3/2  "heat_W"
  Constant8/1 -> ThermalSink3/1, Bus Creator4/1  "heat_W"

== system PowerFlowLib2013amdl/Energy & Power Systems/Additional Systems/External Lights ==
  Mission : Inport
  (1-pf)/pf : Gain  Gain=(1-pf_oven)/(pf_oven+eps)
  (1-pf)/pf1 : Gain  Gain=(1-pf_bev)/(pf_bev+eps)
  Bus Creator : BusCreator  Inputs=2
  Bus Creator1 : BusCreator  Inputs=2
  Bus Creator2 : BusCreator  Inputs=5
  Bus Creator3 : BusCreator  Inputs=1
  Bus Creator4 : BusCreator  Inputs=1
  Bus Creator5 : BusCreator  Inputs=1
  Bus Selector : BusSelector  OutputSignals=GalleyOvens_on/off
  Bus Selector1 : BusSelector  OutputSignals=GalleyBev_on/off
  Bus Selector2 : BusSelector  OutputSignals=ReadingLights_%on
  Bus Selector3 : BusSelector  OutputSignals=CabinLights_%on
  Bus Selector4 : BusSelector  OutputSignals=IFEmodules_%on
  Constant : Constant  Value=n_oven*pwr_oven
  Constant1 : Constant  Value=n_bev*pwr_bev
  Constant2 : Constant  Value=n_rlghts * pwr_rlghts
  Constant3 : Constant  Value=n_alghts * pwr_alghts
  Constant4 : Constant  Value=n_IFE * pwr_IFE
  Constant5 : Constant  Value=q_oven
  Constant6 : Constant  Value=q_bev
  Constant7 : Constant  Value=q_rlghts
  Constant8 : Constant  Value=q_clghts
  ElectricalSink : PowerFlowLib/Support Functions//Tools/ElectricalSink  Tag=Flow  Description=TwoPhase  load_loc=Cabin  ACDC_load=AC  units=Watts  unq_id=8332
  ElectricalSink1 : PowerFlowLib/Support Functions//Tools/ElectricalSink  Tag=Flow  Description=TwoPhase  load_loc=Cabin  ACDC_load=AC  units=Watts  unq_id=9151
  ElectricalSink2 : PowerFlowLib/Support Functions//Tools/ElectricalSink  Tag=Flow  Description=TwoPhase  load_loc=Cabin  ACDC_load=DC  units=Watts  unq_id=2143
  ElectricalSink3 : PowerFlowLib/Support Functions//Tools/ElectricalSink  Tag=Flow  Description=TwoPhase  load_loc=Cabin  ACDC_load=DC  units=Watts  unq_id=9219
  ElectricalSink4 : PowerFlowLib/Support Functions//Tools/ElectricalSink  Tag=Flow  Description=TwoPhase  load_loc=Cabin  ACDC_load=DC  units=Watts  unq_id=6691
  Product{,1..4} (5 alike) : Product  RndMeth=Zero
  ThermalSink : PowerFlowLib/Support Functions//Tools/ThermalSink  Tag=Flow  Description=TwoPhase  load_loc=Cabin  units=Watts  unq_id=1878
  ThermalSink1 : PowerFlowLib/Support Functions//Tools/ThermalSink  Tag=Flow  Description=TwoPhase  load_loc=Cabin  units=Watts  unq_id=3506
  ThermalSink2 : PowerFlowLib/Support Functions//Tools/ThermalSink  Tag=Flow  Description=TwoPhase  load_loc=Cabin  units=Watts  unq_id=5921
  ThermalSink3 : PowerFlowLib/Support Functions//Tools/ThermalSink  Tag=Flow  Description=TwoPhase  load_loc=Cabin  units=Watts  unq_id=9617
  data_sink : PowerFlowLib/Support Functions//Tools/data_sink
  wires:
  Constant8/1 -> ThermalSink3/1
  Constant7/1 -> ThermalSink2/1
  Constant6/1 -> ThermalSink1/1
  Constant5/1 -> ThermalSink/1
  Bus Creator5/1 -> Bus Creator2/5  "IFE"
  Bus Creator4/1 -> Bus Creator2/4  "CabLights"
  Bus Creator3/1 -> Bus Creator2/3  "ReadLights"
  Bus Creator1/1 -> Bus Creator2/2  "Bev_Makers"
  Bus Creator/1 -> Bus Creator2/1  "Ovens"
  Bus Creator2/1 -> data_sink/1
  Bus Selector/1 -> Product/2  "<GalleyOvens_on/off>"
  Bus Selector1/1 -> Product1/2  "<GalleyBev_on/off>"
  Bus Selector2/1 -> Product2/2  "<ReadingLights_%on>"
  Bus Selector3/1 -> Product3/2  "<CabinLights_%on>"
  Bus Selector4/1 -> Product4/2  "<IFEmodules_%on>"
  Mission/1 -> Bus Selector3/1, Bus Selector4/1, Bus Selector2/1, Bus Selector1/1, Bus Selector/1
  Product4/1 -> Bus Creator5/1, ElectricalSink4/1  "pwr_W"
  Constant4/1 -> Product4/1
  Product3/1 -> Bus Creator4/1, ElectricalSink3/1  "pwr_W"
  Constant3/1 -> Product3/1
  Product2/1 -> Bus Creator3/1, ElectricalSink2/1  "pwr_W"
  Constant2/1 -> Product2/1
  Product1/1 -> Bus Creator1/1, ElectricalSink1/1, (1-pf)/pf1/1  "real_pwr_W"
  Constant1/1 -> Product1/1
  (1-pf)/pf1/1 -> Bus Creator1/2, ElectricalSink1/2  "react_pwr_VAr"
  Product/1 -> Bus Creator/1, ElectricalSink/1, (1-pf)/pf/1  "real_pwr_W"
  Constant/1 -> Product/1
  (1-pf)/pf/1 -> Bus Creator/2, ElectricalSink/2  "react_pwr_VAr"

== system PowerFlowLib2013amdl/Energy & Power Systems/Electrical/Battery ==
  note: Battery Model
  BATTERY : Subsystem  AncestorBlock=PowerFlowLib/Energy & Power Systems/Electrical/Battery/BATTERY 10//10  mask{NO_CELLS=9, NO_MODULES=10, INITIAL_SOC=1}
      mask prompts: NO_CELLS "Number of cells in each module"; NO_MODULES "Number of modules"; INITIAL_SOC "Initial SOC"
      mask Display:
      | image(imread('Battery.png'))
      | 
      | port_label('input',1,'{\bf CTOUT}','TexMode','on')
      | port_label('input',2,'{\bf CTIN}','TexMode','on')
      | 
      | port_label('output',1,'{\bf VDC}','TexMode','on')
      | port_label('output',2,'{\bf PLOSS}','TexMode','on')

== system PowerFlowLib2013amdl/Energy & Power Systems/Electrical/Converters ==
  note: Converters
  Boost converter (CCM only; ideal averaged) : Subsystem  mask(Boost converter (Basic averaged model).){L=10e-6, C=100e-6}
      mask prompts: L "Inductance (H):"; C "Output capacitance (F):"
      mask help: Basic boost converter. Lossless storage elements. Averaged model.
  Buck converter (CCM only; ideal averaged) : Subsystem  mask(Buck converter (Basic averaged model).){L=100e-6, C=100e-6}
      mask prompts: L "Inductance (H):"; C "Output capacitance (F):"
      mask help: Basic buck converter. Lossless storage elements. Averaged model.
  Buck-boost converter   (CCM only; ideal averaged) : Subsystem  mask(Buck-boost converter (Basic averaged model).){L=10e-6, C=100e-6}
      mask prompts: L "Inductance (H):"; C "Output capacitance (F):"
      mask help: Basic buck-boost converter. Lossless storage elements. Averaged model.
  Chopper (Averaged) : Subsystem  mask(Chopper.){}
      mask help: Basic chopper. Lossless storage elements. Switching model.
  Chopper (Averaged)1 : Subsystem  mask(Chopper.){}
      mask help: Basic chopper. Lossless storage elements. Switching model.
  rectifier : Subsystem  mask{L=1e-1}
      mask prompts: L "Inductance"

== system PowerFlowLib2013amdl/Energy & Power Systems/Electrical/Coordinate Transformation ==
  note: Coordinate Transformation
  abc to qd0 : Subsystem
      mask help: abc to qd0 Transform.
  qd0 to abc : Subsystem
      mask help: qd0 to abc Transform.
  qde to qds : Subsystem
      mask help: Arbitrary Reference Frame Transform.

== system PowerFlowLib2013amdl/Energy & Power Systems/Electrical/Inverters ==
  note: Voltage Source Inverter
  note: Current Source Inverter
  " inverter" : Subsystem  mask(Average inverter model){Trise=4e-6, Tfall=4e-6, fsw=2e3, Vcesat=1.2, Nofsw=6}
      mask prompts: Trise "Switch rise time (s)"; Tfall "Switch fall time (s)"; fsw "Switching frequency"; Vcesat "Switch vCE on-state voltage"; Nofsw "Number of switches"
      mask help:
      | Inputs
      | #1: qd0 Switching signal
      | #2: DC Voltage [V]
      | #3: Current [A qd0]
      |
      | Outputs
      | #1: Voltage [V qd0]
      | #2: DC Current [A]
      | #3: Power Loss [W]
      mask Display:
      | image(imread('Inverter.png'))
      | port_label('input',1,'{\bf q_q_d_0}','TexMode','on')
      | port_label('input',2,'{\bf V_D_C}','TexMode','on')
      | port_label('input',3,'{\bf I_q_d_0}','TexMode','on')
      | 
      | 
      | port_label('output',1,'{\bf V_q_d_0}','TexMode','on')
      | port_label('output',2,'{\bf I_D_C}','TexMode','on')
      | port_label('output',3,'{\bf P_l_o_s_s}','TexMode','on')
  1phs Inverter (2-level) - average : Subsystem  mask(Single-phase two-level PWM inverter. (Averaged model.)){}
      mask help: Single-phase two-level PWM inverter. This is the averaged model, hence there is no switching frequency input. The modulation function input m(t) must be between 0 and 1.
  1phs Inverter (2-level) - switching : Subsystem  mask(Single-phase two-level PWM inverter. (Switching model.)){f_s=1e3}
      mask prompts: f_s "Switching frequency (Hz):"
      mask help: Single-phase two-level PWM inverter. Switching frequency is set by double-clicking the block. The modulation function input m(t) must be between 0 and 1.
  Current controller : Subsystem  mask{R_IGBT=0, CR_gain=0, V_IGBT=0}
      mask prompts: R_IGBT "IGBT On-state Resistance"; CR_gain "Current Regulator Gain"; V_IGBT "IGBT Saturation Voltage"
      mask help: Current Control.
      mask Display:
      | plot([0 0], [0.3 -0.3])
      | port_label('output',1,'va')
      | port_label('output',2,'vb')
      | port_label('output',3,'vc')
      | port_label('input',1,'ia*')
      | port_label('input',2,'ib*')
      | port_label('input',3,'ic*')
      | port_label('input',4,'ia')
      | port_label('input',5,'ib')
      | port_label('input',6,'ic')
      | port_label('input',7,'V_bus')
  Inverter (Average) : Subsystem  mask{Freq=0}
      mask prompts: Freq "Switching Frequency"
      mask help: Average inverter model (Please input the switching frequency)
  Inverter (Switching  Model) - Current  Control : Subsystem
      mask help:
      | Switched inverter model.
      | Hysteretic current control.
  three-phase  full-bridge  inverter : Subsystem
      mask help:
      | Three-phase full bridge inverter:
      | INPUTS:
      | - three phase binary switching fucntions (qa, qb, qc)
      | - dc bus voltage Vdc [V]
      | - output phase currents (ia,ib,ic) [A]
      |
      | OUPTUTS:
      | - dc bus input current (Idc) [A]
      | - inverter line-to-line voltages (Vab, Vbc, Vca) [V]
  three-phase  full-bridge  inverter1 : Subsystem
      mask help: 3 phase full bridge inverter

== system PowerFlowLib2013amdl/Energy & Power Systems/Electrical/Loads ==
  note: Electrical Loads
  Constant Current Load : Subsystem
      mask help: Constant Current Load.
  Constant Power Load : Subsystem
      mask help: Constant Power Load.
  Enabled  DC Load1 : Subsystem
      mask help: Enabled DC Load System.
  Enabled_AC_Loadloss : Subsystem  mask{P=500, PF=0.85, E=0.98, ILRMS=0, R=10000, X=10000}
      mask prompts: P "Real Power (W)"; PF "Power factor (Range: 0 -1) : Prefix '-' sign for Cap loads"; E "Load Efficiency (Range: 0 - 1)"; ILRMS "Current Loading"; R "Resistance (Ohms)"; X "Reactance (Ohms)"
      mask help:
      | Enabled AC Load System.
      | Note:
      | Load Master Vector input is 1x3 matrix representing (P[W] Q[Var] I[A])
      | Extra load can be input in the boxes below and will be added with the Load Master Vector.
      mask Callback PF:
      | blk = gcb;
      | PF    = str2num(get_param(blk,'PF'));
      | 
      | if ((PF>1) | (PF<-1))
      |    g = warndlg('Power factor magnitude should be between 0 and 1 . Reverting to default value 1','Error1','CreateMode');
      |    set_param(blk,'PF','1');
      |    open_system(blk,'mask');
      | end
      | 
      | clear g PF blk
      mask Callback E:
      | blk = gcb;
      | eff    = str2num(get_param(blk,'E'));
      | 
      | if ((eff>1) | (eff<0))
      |    g = warndlg('Efficiency should be between 0 and 1 . Reverting to default value 1','Error1','CreateMode');
      |    set_param(blk,'E','1');
      |    open_system(blk,'mask');
      | end
      | 
      | clear g eff blk
      mask Callback X:
      | blk = gcb;
      | value1 = str2num(get_param(blk,'R'));
      | value2 = str2num(get_param(blk,'X'));
      | % eff    = str2num(get_param(blk,'E'));
      | 
      | if (value1==0) && (value2==0)
      |   h = warndlg('Both R and X cannot be 0. Reverting to default values','Error','CreateMode');
      |   set_param(blk,'R','10000');
      |   set_param(blk,'X','10000');
      | %   if ishandle(h)
      | %       close(h)
      |   open_system(blk,'mask');
      | end
      | 
      | % if ((eff>1) | (eff<0))
      | %    g = warndlg('Efficiency should be between 0 and 1 . Reverting to default value 1','Error1','CreateMode');
      | %    set_param(blk,'E','1');
      | %    open_system(blk,'mask');
      | % end
      | 
      | clear h eff blk value1 value2
      mask Display:
      | %image(imread('ACload.png'))
      | 
      | % port_label('input',1,'{\bf EXT LOAD VECTOR}','TexMode','on')
      | % port_label('input',2,'{\bf Vdq0}','TexMode','on')
      | %
      | % port_label('output',1,'{\bf Idq0}','TexMode','on')
      | % port_label('output',2,'{\bf PLOSS}','TexMode','on')

== system PowerFlowLib2013amdl/Energy & Power Systems/Electrical/Loss Estimation ==
  note: Power Loss Estimation
  DC/DC Converter - Boost : Subsystem
      mask help: Power Loss Estimation block for a Boost Converter.
  DC/DC Converter - Buck : Subsystem
      mask help: Power Loss Estimation block for a Buck Converter.
  Three-Phase ACTIVE RECTIFIER : Subsystem
      mask help: Power Loss Estimation block for an active rectifier.
  Three-Phase Diode Full Bridge  PASSIVE RECTIFIER : Subsystem
      mask help: Power Loss Estimation block for a 3 phase full bridge rectifier.
  Three-Phase Full Bridge Inverter CONSTANT FREQUENCY : Subsystem
      mask help: Power Loss Estimation block for a 3 phase full bridge constant frequency inverter.
  Three-Phase Full Bridge Inverter VARIABLE FREQUENCY : Subsystem
      mask help: Power Loss Estimation block for a 3 phase full bridge variable frequency inverter.
